simulink model "tpi2series2parallel"  (R2017b)
settings: Solver=ode8  StartTime=0.0  StopTime=0.1  FixedStep=1e-6  MaxStep=1e-4  RelTol=1e-3
values from neighbouring files (symbols this model uses):
  dcin = 547.66    [tpi2parallelrunner.m]    (also in tpi2seriesrunner.m; tpireloadedrunner.m)
  Ef = 154.55/2    (= 77.275)    [tpi2seriesrunner.m]    (also in tpireloadedrunner.m)
  fdclinkcap = 100e-6    (= 0.0001)    [tpi2parallelrunner.m]    (also in tpi2seriesrunner.m; tpireloadedrunner.m = 0.01)
  fdclinkres = 1e-6    (= 1e-06)    [tpi2parallelrunner.m]    (also in tpi2seriesrunner.m; tpireloadedrunner.m)
  FLload = FXload/freffreq    [tpi2parallelrunner.m]    (also in tpi2seriesrunner.m; tpireloadedrunner.m)
  fma = 0.9    [tpi2parallelrunner.m]    (also in tpi2seriesrunner.m; tpireloadedrunner.m)
  freffreq = 2*pi*50    (= 314.159265359)    [tpi2parallelrunner.m]    (also in tpi2seriesrunner.m; tpireloadedrunner.m)
  FRload = FZload*Load_Power_Factor    [tpi2parallelrunner.m]    (also in tpi2seriesrunner.m = n*FZload*Load_Power_Factor; tpireloadedrunner.m = n*FZload*Load_Power_Factor)
  Rin = 1    [tpi2parallelrunner.m]    (also in tpi2seriesrunner.m; tpireloadedrunner.m)
  sdclinkcap = 100e-6    (= 0.0001)    [tpi2seriesrunner.m]    (also in tpireloadedrunner.m = 0.01)
  sdclinkres = 1e-6    (= 1e-06)    [tpi2seriesrunner.m]    (also in tpireloadedrunner.m)
  SLload = SXload/sreffreq    [tpi2parallelrunner.m]    (also in tpi2seriesrunner.m; tpireloadedrunner.m)
  sma = 0.9    [tpi2parallelrunner.m]    (also in tpi2seriesrunner.m; tpireloadedrunner.m)
  sreffreq = 2*pi*50    (= 314.159265359)    [tpi2parallelrunner.m]    (also in tpi2seriesrunner.m; tpireloadedrunner.m)
  SRload = SZload*Load_Power_Factor    [tpi2parallelrunner.m]    (also in tpi2seriesrunner.m = n*SZload*Load_Power_Factor; tpireloadedrunner.m = n*SZload*Load_Power_Factor)
undefined symbols (not defined in the file or in its folder): fdclink1cap
libraries: powerlib x82, simulink x12, powerlib_meascontrol x10, dspstat3 x9
settings Model: Creator=Orhun  LastModifiedBy=Orhun
settings SolverCC: ZeroCrossAlgorithm=Adaptive
settings DebuggingCC: MaxConsecutiveZCsMsg=none

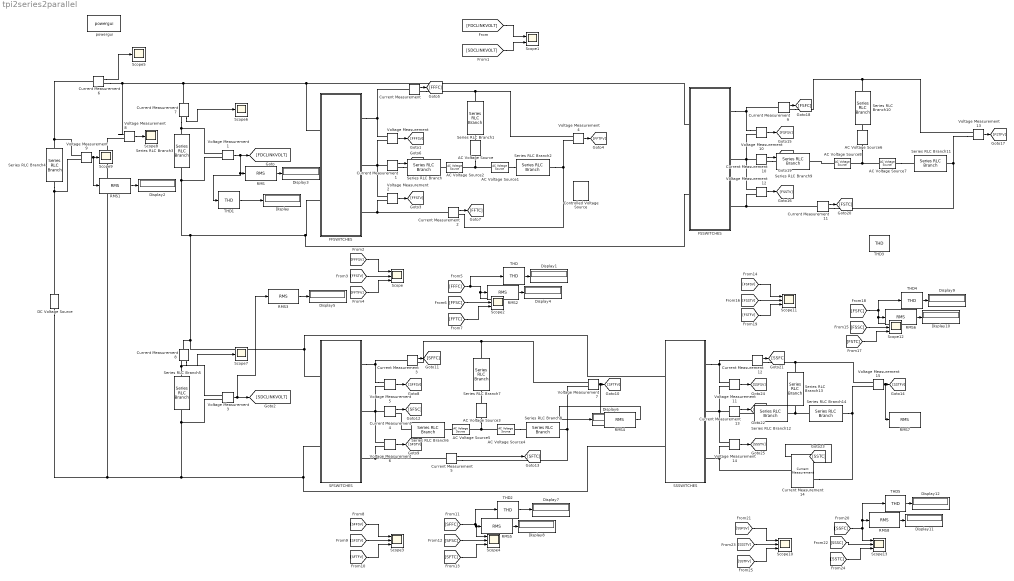
== system tpi2series2parallel ==
  AC Voltage Source : powerlib/Electrical Sources/AC Voltage Source  Amplitude=Ef*sqrt(2)  Phase=0  Frequency=freffreq  SampleTime=0  Measurements=None  BusType=swing  Pref=10e3  Qref=0  Qmin=-inf  Qmax=+inf
  AC Voltage Source1 : powerlib/Electrical Sources/AC Voltage Source  Amplitude=Ef*sqrt(2)  Phase=-2*pi/3  Frequency=freffreq  SampleTime=0  Measurements=None  BusType=swing  Pref=10e3  Qref=0  Qmin=-inf  Qmax=+inf
  AC Voltage Source2 : powerlib/Electrical Sources/AC Voltage Source  Amplitude=Ef*sqrt(2)  Phase=2*pi/3  Frequency=freffreq  SampleTime=0  Measurements=None  BusType=swing  Pref=10e3  Qref=0  Qmin=-inf  Qmax=+inf
  AC Voltage Source3 : powerlib/Electrical Sources/AC Voltage Source  Amplitude=Ef*sqrt(2)  Phase=0  Frequency=sreffreq  SampleTime=0  Measurements=None  BusType=swing  Pref=10e3  Qref=0  Qmin=-inf  Qmax=+inf
  AC Voltage Source4 : powerlib/Electrical Sources/AC Voltage Source  Amplitude=Ef*sqrt(2)  Phase=-2*pi/3  Frequency=sreffreq  SampleTime=0  Measurements=None  BusType=swing  Pref=10e3  Qref=0  Qmin=-inf  Qmax=+inf
  AC Voltage Source5 : powerlib/Electrical Sources/AC Voltage Source  Amplitude=Ef*sqrt(2)  Phase=2*pi/3  Frequency=sreffreq  SampleTime=0  Measurements=None  BusType=swing  Pref=10e3  Qref=0  Qmin=-inf  Qmax=+inf
  AC Voltage Source6 : powerlib/Electrical Sources/AC Voltage Source  Amplitude=Ef*sqrt(2)  Phase=0  Frequency=freffreq  SampleTime=0  Measurements=None  BusType=swing  Pref=10e3  Qref=0  Qmin=-inf  Qmax=+inf
  AC Voltage Source7 : powerlib/Electrical Sources/AC Voltage Source  Amplitude=Ef*sqrt(2)  Phase=-2*pi/3  Frequency=freffreq  SampleTime=0  Measurements=None  BusType=swing  Pref=10e3  Qref=0  Qmin=-inf  Qmax=+inf
  AC Voltage Source8 : powerlib/Electrical Sources/AC Voltage Source  Amplitude=Ef*sqrt(2)  Phase=2*pi/3  Frequency=freffreq  SampleTime=0  Measurements=None  BusType=swing  Pref=10e3  Qref=0  Qmin=-inf  Qmax=+inf
  Controlled Voltage Source : powerlib/Electrical Sources/Controlled Voltage Source  Initialize=on  Source_Type=AC  Amplitude=0  Phase=0  Frequency=0  Measurements=None
  Current Measurement{,1..14} (15 alike) : powerlib/Measurements/Current Measurement  PhasorSimulation=off  OutputType=Complex  PSBequivalent=0
  DC Voltage Source : powerlib/Electrical Sources/DC Voltage Source  Amplitude=dcin  Measurements=None
  Display{,1..12} (13 alike) : Display
  FFSWITCHES : Subsystem
  FSSWITCHES : Subsystem
  RMS : dspstat3/RMS  run=on  directionMode=Each column  dimension=1  InputProcessing=Columns as channels (frame based)  reset_popup=None
  RMS1 : dspstat3/RMS  run=off  directionMode=Each column  dimension=1  InputProcessing=Columns as channels (frame based)  reset_popup=None
  RMS{2,4..8} (6 alike) : dspstat3/RMS  run=on  directionMode=Entire input  dimension=1  InputProcessing=Columns as channels (frame based)  reset_popup=None
  RMS3 : dspstat3/RMS  run=off  directionMode=Each column  dimension=1  InputProcessing=Columns as channels (frame based)  reset_popup=None
  SFSWITCHES : Subsystem
  SSSWITCHES : Subsystem
  Scope{,2..4,10..13} (8 alike) : Scope  NumInputPorts=3
  Scope1 : Scope  NumInputPorts=2
  Scope{5..9} (5 alike) : Scope
  Series RLC Branch{,1..2,9..11} (6 alike) : powerlib/Elements/Series RLC Branch  LConnTagsString=__new0  RConnTagsString=__new0  BranchType=RL  Resistance=FRload  Inductance=FLload  SetiL0=off  InitialCurrent=0  Capacitance=0  Setx0=off  InitialVoltage=0  Measurements=None
  Series RLC Branch{6..8,12..14} (6 alike) : powerlib/Elements/Series RLC Branch  LConnTagsString=__new0  RConnTagsString=__new0  BranchType=RL  Resistance=SRload  Inductance=SLload  SetiL0=off  InitialCurrent=0  Capacitance=0  Setx0=off  InitialVoltage=0  Measurements=None
  Series RLC Branch3 : powerlib/Elements/Series RLC Branch  LConnTagsString=__new0  RConnTagsString=__new0  BranchType=C  Resistance=fdclinkres  Inductance=0  SetiL0=off  InitialCurrent=0  Capacitance=fdclinkcap  Setx0=off  InitialVoltage=dcin/2  Measurements=None
  Series RLC Branch4 : powerlib/Elements/Series RLC Branch  LConnTagsString=__new0  RConnTagsString=__new0  BranchType=R  Resistance=Rin  Inductance=0  SetiL0=off  InitialCurrent=0  Capacitance=fdclink1cap  Setx0=off  InitialVoltage=0  Measurements=None
  Series RLC Branch5 : powerlib/Elements/Series RLC Branch  LConnTagsString=__new0  RConnTagsString=__new0  BranchType=C  Resistance=sdclinkres  Inductance=0  SetiL0=off  InitialCurrent=0  Capacitance=sdclinkcap  Setx0=off  InitialVoltage=dcin/2  Measurements=None
  THD{,1..5} (6 alike) : powerlib_meascontrol/Measurements/THD  Freq=50  Ts=0
  Voltage Measurement{,1..15} (16 alike) : powerlib/Measurements/Voltage Measurement  PhasorSimulation=off  OutputType=Complex  PSBequivalent=0
  powergui : powerlib/powergui  Priority=1  SimulationMode=Discrete  SampleTime=1e-6  frequency=60  Iterations=50  frequencyindice=0  Pbase=100e6  ErrMax=1e-4  UnitsV=kV  UnitsW=MW  buscounter=0  FunctionMessages=on  echomessages=off  EnableUseOfTLC=off  CurrentSourceSwitches=off  DisableSnubberDevices=off  DisableRonSwitches=off  DisableVfSwitches=off  DisplayEquations=off  SolverType=Tustin/Backward Euler (TBE)  Interpol=off  ExternalGateDelay=off  methode=off  Ts=100  x0status=blocks  SPID=off  SwTol=0  HookPort=off  RestoreLinks=warning  ResistiveCurrentMeasurement=off  Frange=[0:2:500]  Ylog=off  Xlog=on  ShowGrid=off  save=off  variable=ZData  structure=0  ZoomFFT=off  StartTime=0.0  cycles=1  DisplayStyle=1  fundamental=60  FreqAxis=off  MaxFrequency=1000  frequencyindicesteady=1  RmsSteady=1  display=off
  wires:
  Voltage Measurement1/1 -> RMS/1, THD1/1, [FDCLINKVOLT]
  Voltage Measurement3/1 -> RMS3/1, [SDCLINKVOLT]
  [FDCLINKVOLT] -> Scope1/1
  [SDCLINKVOLT] -> Scope1/2
  Voltage Measurement/1 -> [FFFSV]
  Voltage Measurement2/1 -> [FFSTV]
  Voltage Measurement4/1 -> [FFTFV]
  Current Measurement/1 -> [FFFC]
  Current Measurement1/1 -> [FFSC]
  Current Measurement2/1 -> [FFTC]
  [FFFSV] -> Scope/1
  [FFSTV] -> Scope/2
  [FFTFV] -> Scope/3
  [FFFC] -> THD/1, RMS2/1, Scope2/1
  [SFSTV] -> Scope3/2
  [SFTC] -> Scope4/3
  [SFTFV] -> Scope3/3
  [SFSC] -> Scope4/2
  [SFFSV] -> Scope3/1
  [SFFC] -> THD2/1, RMS5/1, Scope4/1
  Current Measurement3/1 -> [SFFC]
  Current Measurement4/1 -> [SFSC]
  Voltage Measurement5/1 -> [SFFSV]
  Voltage Measurement6/1 -> [SFSTV]
  Current Measurement5/1 -> [SFTC]
  Voltage Measurement7/1 -> RMS4/1, [SFTFV]
  Current Measurement6/1 -> Scope5/1
  THD1/1 -> Display/1
  Current Measurement7/1 -> Scope6/1
  Current Measurement8/1 -> Scope7/1
  THD/1 -> Display1/1
  Voltage Measurement8/1 -> Scope8/1
  Voltage Measurement9/1 -> RMS1/1, Scope9/1
  RMS1/1 -> Display2/1
  RMS/1 -> Display3/1
  RMS2/1 -> Display4/1
  RMS3/1 -> Display5/1
  RMS4/1 -> Display6/1
  [FFSC] -> Scope2/2
  [FFTC] -> Scope2/3
  THD2/1 -> Display7/1
  Current Measurement9/1 -> [FSFC]
  Current Measurement11/1 -> [FSTC]
  Voltage Measurement10/1 -> [FSFSV]
  Current Measurement10/1 -> [FSSC]
  Voltage Measurement13/1 -> [FSTFV]
  Voltage Measurement12/1 -> [FSSTV]
  [FSFSV] -> Scope11/1
  RMS6/1 -> Display10/1
  THD4/1 -> Display9/1
  [FSTC] -> Scope12/3
  [FSFC] -> THD4/1, RMS6/1, Scope12/1
  Voltage Measurement15/1 -> RMS7/1, [SSTFV]
  Voltage Measurement11/1 -> [SSFSV]
  Current Measurement14/1 -> [SSTC]
  Voltage Measurement14/1 -> [SSSTV]
  Current Measurement12/1 -> [SSFC]
  Current Measurement13/1 -> [SSSC]
  [SSFSV] -> Scope10/1
  [SSSTV] -> Scope10/2
  [SSTFV] -> Scope10/3
  [SSSC] -> Scope13/2
  [SSFC] -> RMS8/1, THD5/1, Scope13/1
  RMS8/1 -> Display11/1
  [SSTC] -> Scope13/3
  THD5/1 -> Display12/1
  [FSSC] -> Scope12/2
  [FSTFV] -> Scope11/3
  [FSSTV] -> Scope11/2
  RMS5/1 -> Display8/1
  connections:
  Current Measurement6/RConn1 -- Voltage Measurement8/LConn1 -- Current Measurement7/LConn1 -- FSSWITCHES/LConn1 -- FFSWITCHES/LConn1
  Voltage Measurement1/LConn2 -- FSSWITCHES/LConn2 -- FFSWITCHES/LConn2 -- SSSWITCHES/LConn1 -- SFSWITCHES/LConn1 -- Current Measurement8/LConn1 -- Series RLC Branch3/RConn1
  Series RLC Branch4/RConn1 -- Voltage Measurement9/LConn2 -- DC Voltage Source/RConn1
  Voltage Measurement3/LConn2 -- Voltage Measurement8/LConn2 -- DC Voltage Source/LConn1 -- SSSWITCHES/LConn2 -- SFSWITCHES/LConn2 -- Series RLC Branch5/RConn1
  FFSWITCHES/RConn1 -- Current Measurement/LConn1 -- Voltage Measurement/LConn1
  FFSWITCHES/RConn2 -- Current Measurement1/LConn1 -- Voltage Measurement2/LConn1 -- Voltage Measurement/LConn2
  Series RLC Branch2/LConn1 -- Current Measurement2/RConn1 -- Voltage Measurement4/LConn1
  Current Measurement/RConn1 -- Series RLC Branch1/RConn1 -- Voltage Measurement4/LConn2
  Current Measurement1/RConn1 -- Series RLC Branch/RConn1
  Voltage Measurement2/LConn2 -- Current Measurement2/LConn1 -- FFSWITCHES/RConn3
  Current Measurement3/RConn1 -- Series RLC Branch7/RConn1 -- Voltage Measurement7/LConn2
  Voltage Measurement5/LConn1 -- SFSWITCHES/RConn1 -- Current Measurement3/LConn1
  Voltage Measurement5/LConn2 -- SFSWITCHES/RConn2 -- Current Measurement4/LConn1 -- Voltage Measurement6/LConn1
  Series RLC Branch8/LConn1 -- Voltage Measurement7/LConn1 -- Current Measurement5/RConn1
  Voltage Measurement6/LConn2 -- Current Measurement5/LConn1 -- SFSWITCHES/RConn3
  Series RLC Branch6/RConn1 -- Current Measurement4/RConn1
  Current Measurement6/LConn1 -- Voltage Measurement9/LConn1 -- Series RLC Branch4/LConn1
  Voltage Measurement1/LConn1 -- Current Measurement7/RConn1 -- Series RLC Branch3/LConn1
  Series RLC Branch5/LConn1 -- Voltage Measurement3/LConn1 -- Current Measurement8/RConn1
  FSSWITCHES/RConn3 -- Voltage Measurement12/LConn2 -- Current Measurement11/LConn1
  Voltage Measurement10/LConn1 -- FSSWITCHES/RConn1 -- Current Measurement9/LConn1
  Voltage Measurement13/LConn1 -- Series RLC Branch11/LConn1 -- Current Measurement11/RConn1
  Current Measurement9/RConn1 -- Voltage Measurement13/LConn2 -- Series RLC Branch10/RConn1
  Voltage Measurement10/LConn2 -- FSSWITCHES/RConn2 -- Current Measurement10/LConn1 -- Voltage Measurement12/LConn1
  Current Measurement10/RConn1 -- Series RLC Branch9/RConn1
  Current Measurement12/LConn1 -- Voltage Measurement11/LConn1 -- SSSWITCHES/RConn1
  Current Measurement14/RConn1 -- Voltage Measurement15/LConn1 -- Series RLC Branch14/LConn1
  SSSWITCHES/RConn3 -- Voltage Measurement14/LConn2 -- Current Measurement14/LConn1
  Series RLC Branch12/LConn1 -- Series RLC Branch14/RConn1 -- Series RLC Branch13/LConn1
  Voltage Measurement14/LConn1 -- Voltage Measurement11/LConn2 -- SSSWITCHES/RConn2 -- Current Measurement13/LConn1
  Voltage Measurement15/LConn2 -- Current Measurement12/RConn1 -- Series RLC Branch13/RConn1
  Series RLC Branch12/RConn1 -- Current Measurement13/RConn1
  AC Voltage Source/RConn1 -- Series RLC Branch1/LConn1
  AC Voltage Source1/RConn1 -- Series RLC Branch2/RConn1
  AC Voltage Source2/RConn1 -- Series RLC Branch/LConn1
  AC Voltage Source1/LConn1 -- AC Voltage Source/LConn1 -- AC Voltage Source2/LConn1
  AC Voltage Source4/LConn1 -- AC Voltage Source3/LConn1 -- AC Voltage Source5/LConn1
  AC Voltage Source3/RConn1 -- Series RLC Branch7/LConn1
  Series RLC Branch6/LConn1 -- AC Voltage Source5/RConn1
  AC Voltage Source4/RConn1 -- Series RLC Branch8/RConn1
  AC Voltage Source7/LConn1 -- AC Voltage Source6/LConn1 -- AC Voltage Source8/LConn1
  AC Voltage Source6/RConn1 -- Series RLC Branch10/LConn1
  AC Voltage Source8/RConn1 -- Series RLC Branch9/LConn1
  AC Voltage Source7/RConn1 -- Series RLC Branch11/RConn1

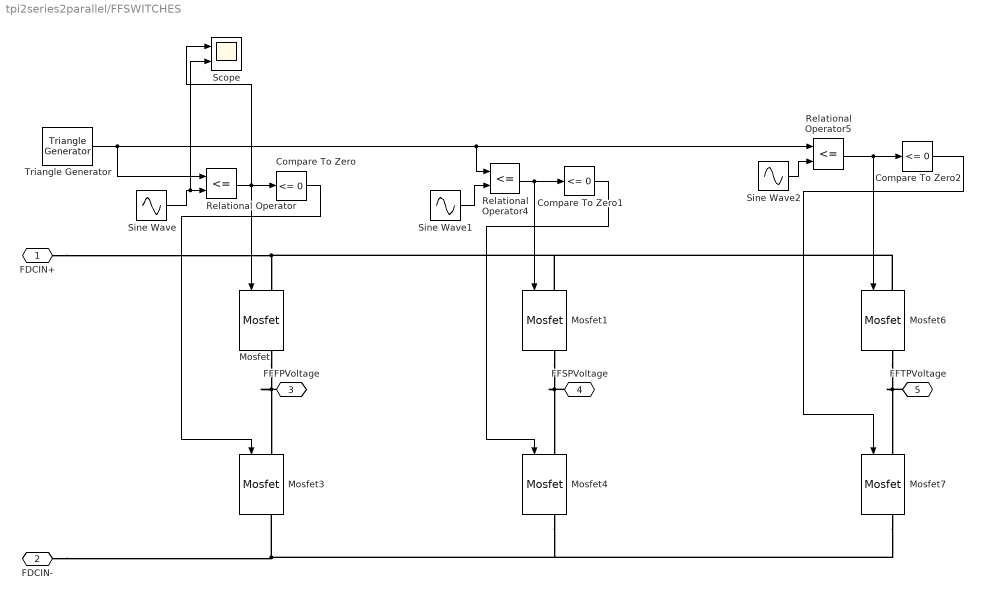
== system tpi2series2parallel/FFSWITCHES ==
  Compare To Zero : simulink/Logic and Bit Operations/Compare To Zero  relop=<=  OutDataTypeStr=boolean
  Compare To Zero1 : simulink/Logic and Bit Operations/Compare To Zero  relop=<=  OutDataTypeStr=boolean
  Compare To Zero2 : simulink/Logic and Bit Operations/Compare To Zero  relop=<=  OutDataTypeStr=boolean
  Mosfet{,1,3..4,6..7} (6 alike) : powerlib/Power Electronics/Mosfet  Ron=2e-3  Lon=0  Rd=0.01  Vfd=0  IC=0  Rs=1e5  Cs=inf  Measurements=on
  Relational Operator : RelationalOperator  Operator=<=  OutDataTypeStr=boolean  RndMeth=Simplest
  Relational Operator4 : RelationalOperator  Operator=<=  OutDataTypeStr=boolean  RndMeth=Simplest
  Relational Operator5 : RelationalOperator  Operator=<=  OutDataTypeStr=boolean  RndMeth=Simplest
  Scope : Scope  NumInputPorts=2
  Sine Wave : Sin  Amplitude=fma  Frequency=freffreq  SampleTime=0
  Sine Wave1 : Sin  Amplitude=fma  Frequency=freffreq  Phase=2*pi/3  SampleTime=0
  Sine Wave2 : Sin  Amplitude=fma  Frequency=freffreq  Phase=4*pi/3  SampleTime=0
  Triangle Generator : powerlib_meascontrol/Pulse & Signal Generators/Triangle Generator  Freq=fswfreq  Phase=90  Ts=1e-6
  FDCIN+ : PMIOPort  Port=1  Side=Left
  FDCIN- : PMIOPort  Port=2  Side=Left
  FFFPVoltage : PMIOPort  Port=3  Side=Right
  FFSPVoltage : PMIOPort  Port=4  Side=Right
  FFTPVoltage : PMIOPort  Port=5  Side=Right
  wires:
  Sine Wave/1 -> Scope/2, Relational Operator/2
  Triangle Generator/1 -> Relational Operator5/1, Relational Operator4/1, Relational Operator/1
  Relational Operator4/1 -> Mosfet1/1, Compare To Zero1/1
  Sine Wave2/1 -> Relational Operator5/2
  Sine Wave1/1 -> Relational Operator4/2
  Relational Operator/1 -> Mosfet/1, Scope/1, Compare To Zero/1
  Compare To Zero/1 -> Mosfet3/1
  Compare To Zero1/1 -> Mosfet4/1
  Compare To Zero2/1 -> Mosfet7/1
  Relational Operator5/1 -> Mosfet6/1, Compare To Zero2/1
  connections:
  Mosfet6/RConn1 -- FFTPVoltage/RConn1 -- Mosfet7/LConn1
  Mosfet/RConn1 -- FFFPVoltage/RConn1 -- Mosfet3/LConn1
  Mosfet1/RConn1 -- FFSPVoltage/RConn1 -- Mosfet4/LConn1
  FDCIN+/RConn1 -- Mosfet6/LConn1 -- Mosfet1/LConn1 -- Mosfet/LConn1
  FDCIN-/RConn1 -- Mosfet4/RConn1 -- Mosfet7/RConn1 -- Mosfet3/RConn1

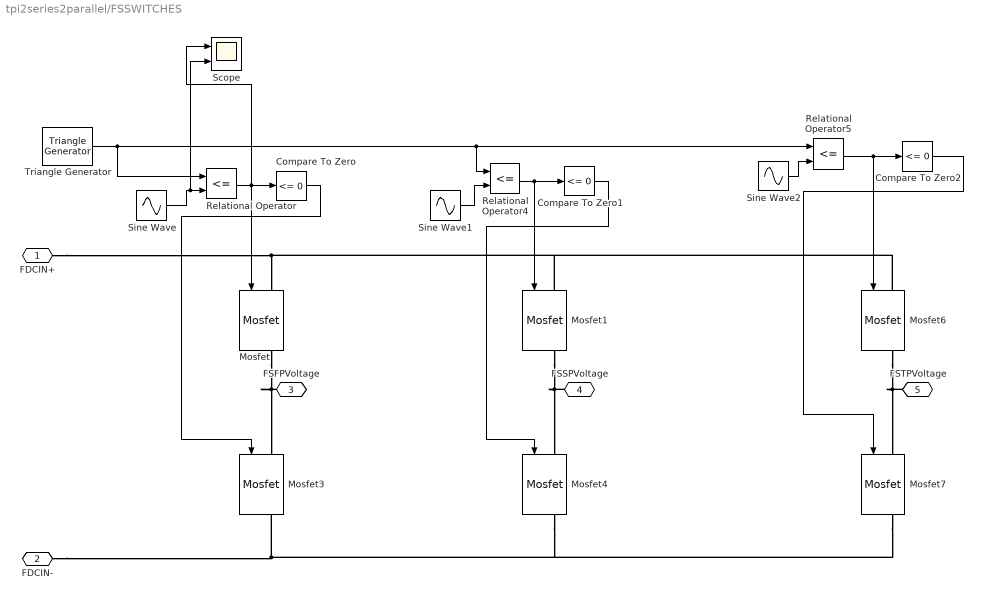
== system tpi2series2parallel/FSSWITCHES ==
  Compare To Zero : simulink/Logic and Bit Operations/Compare To Zero  relop=<=  OutDataTypeStr=boolean
  Compare To Zero1 : simulink/Logic and Bit Operations/Compare To Zero  relop=<=  OutDataTypeStr=boolean
  Compare To Zero2 : simulink/Logic and Bit Operations/Compare To Zero  relop=<=  OutDataTypeStr=boolean
  Mosfet{,1,3..4,6..7} (6 alike) : powerlib/Power Electronics/Mosfet  Ron=2e-3  Lon=0  Rd=0.01  Vfd=0  IC=0  Rs=1e5  Cs=inf  Measurements=on
  Relational Operator : RelationalOperator  Operator=<=  OutDataTypeStr=boolean  RndMeth=Simplest
  Relational Operator4 : RelationalOperator  Operator=<=  OutDataTypeStr=boolean  RndMeth=Simplest
  Relational Operator5 : RelationalOperator  Operator=<=  OutDataTypeStr=boolean  RndMeth=Simplest
  Scope : Scope  NumInputPorts=2
  Sine Wave : Sin  Amplitude=fma  Frequency=freffreq  SampleTime=0
  Sine Wave1 : Sin  Amplitude=fma  Frequency=freffreq  Phase=2*pi/3  SampleTime=0
  Sine Wave2 : Sin  Amplitude=fma  Frequency=freffreq  Phase=4*pi/3  SampleTime=0
  Triangle Generator : powerlib_meascontrol/Pulse & Signal Generators/Triangle Generator  Freq=fswfreq  Phase=90  Ts=1e-6
  FDCIN+ : PMIOPort  Port=1  Side=Left
  FDCIN- : PMIOPort  Port=2  Side=Left
  FSFPVoltage : PMIOPort  Port=3  Side=Right
  FSSPVoltage : PMIOPort  Port=4  Side=Right
  FSTPVoltage : PMIOPort  Port=5  Side=Right
  wires:
  Sine Wave/1 -> Scope/2, Relational Operator/2
  Triangle Generator/1 -> Relational Operator5/1, Relational Operator4/1, Relational Operator/1
  Relational Operator4/1 -> Mosfet1/1, Compare To Zero1/1
  Sine Wave2/1 -> Relational Operator5/2
  Sine Wave1/1 -> Relational Operator4/2
  Relational Operator/1 -> Mosfet/1, Scope/1, Compare To Zero/1
  Compare To Zero/1 -> Mosfet3/1
  Compare To Zero1/1 -> Mosfet4/1
  Compare To Zero2/1 -> Mosfet7/1
  Relational Operator5/1 -> Mosfet6/1, Compare To Zero2/1
  connections:
  Mosfet6/RConn1 -- FSTPVoltage/RConn1 -- Mosfet7/LConn1
  Mosfet/RConn1 -- FSFPVoltage/RConn1 -- Mosfet3/LConn1
  Mosfet1/RConn1 -- FSSPVoltage/RConn1 -- Mosfet4/LConn1
  FDCIN+/RConn1 -- Mosfet6/LConn1 -- Mosfet1/LConn1 -- Mosfet/LConn1
  FDCIN-/RConn1 -- Mosfet4/RConn1 -- Mosfet7/RConn1 -- Mosfet3/RConn1

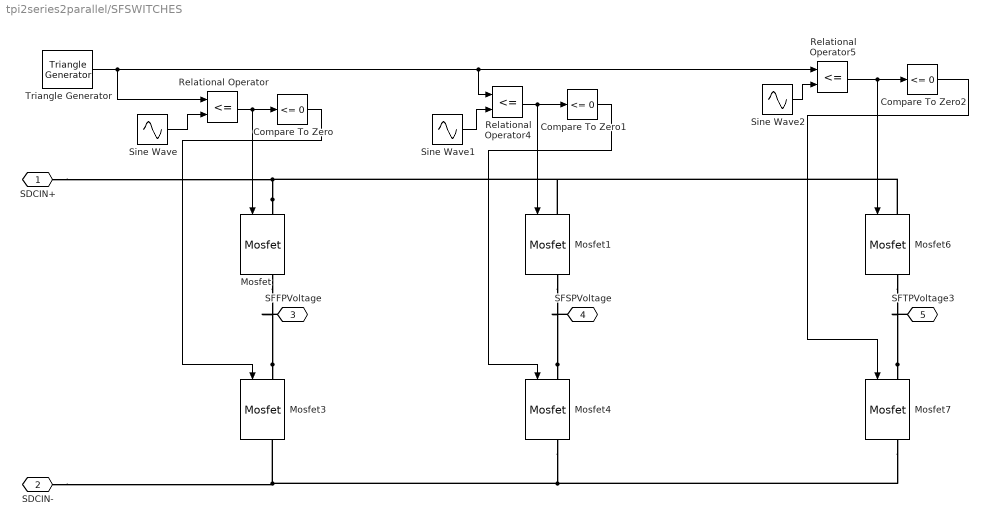
== system tpi2series2parallel/SFSWITCHES ==
  Compare To Zero : simulink/Logic and Bit Operations/Compare To Zero  relop=<=  OutDataTypeStr=boolean
  Compare To Zero1 : simulink/Logic and Bit Operations/Compare To Zero  relop=<=  OutDataTypeStr=boolean
  Compare To Zero2 : simulink/Logic and Bit Operations/Compare To Zero  relop=<=  OutDataTypeStr=boolean
  Mosfet{,1,3..4,6..7} (6 alike) : powerlib/Power Electronics/Mosfet  Ron=2e-3  Lon=0  Rd=0.01  Vfd=0  IC=0  Rs=1e5  Cs=inf  Measurements=on
  Relational Operator : RelationalOperator  Operator=<=  OutDataTypeStr=boolean  RndMeth=Simplest
  Relational Operator4 : RelationalOperator  Operator=<=  OutDataTypeStr=boolean  RndMeth=Simplest
  Relational Operator5 : RelationalOperator  Operator=<=  OutDataTypeStr=boolean  RndMeth=Simplest
  Sine Wave : Sin  Amplitude=sma  Frequency=sreffreq  SampleTime=0
  Sine Wave1 : Sin  Amplitude=sma  Frequency=sreffreq  Phase=2*pi/3  SampleTime=0
  Sine Wave2 : Sin  Amplitude=fma  Frequency=sreffreq  Phase=4*pi/3  SampleTime=0
  Triangle Generator : powerlib_meascontrol/Pulse & Signal Generators/Triangle Generator  Freq=sswfreq  Phase=270  Ts=1e-6
  SDCIN+ : PMIOPort  Port=1  Side=Left
  SDCIN- : PMIOPort  Port=2  Side=Left
  SFFPVoltage : PMIOPort  Port=3  Side=Right
  SFSPVoltage : PMIOPort  Port=4  Side=Right
  SFTPVoltage3 : PMIOPort  Port=5  Side=Right
  wires:
  Sine Wave/1 -> Relational Operator/2
  Triangle Generator/1 -> Relational Operator5/1, Relational Operator4/1, Relational Operator/1
  Relational Operator4/1 -> Mosfet1/1, Compare To Zero1/1
  Sine Wave2/1 -> Relational Operator5/2
  Sine Wave1/1 -> Relational Operator4/2
  Relational Operator/1 -> Compare To Zero/1, Mosfet/1
  Compare To Zero/1 -> Mosfet3/1
  Compare To Zero1/1 -> Mosfet4/1
  Compare To Zero2/1 -> Mosfet7/1
  Relational Operator5/1 -> Mosfet6/1, Compare To Zero2/1
  connections:
  Mosfet7/LConn1 -- Mosfet6/RConn1 -- SFTPVoltage3/RConn1
  Mosfet3/LConn1 -- Mosfet/RConn1 -- SFFPVoltage/RConn1
  Mosfet4/LConn1 -- Mosfet1/RConn1 -- SFSPVoltage/RConn1
  Mosfet/LConn1 -- SDCIN+/RConn1 -- Mosfet6/LConn1 -- Mosfet1/LConn1
  Mosfet4/RConn1 -- Mosfet3/RConn1 -- SDCIN-/RConn1 -- Mosfet7/RConn1

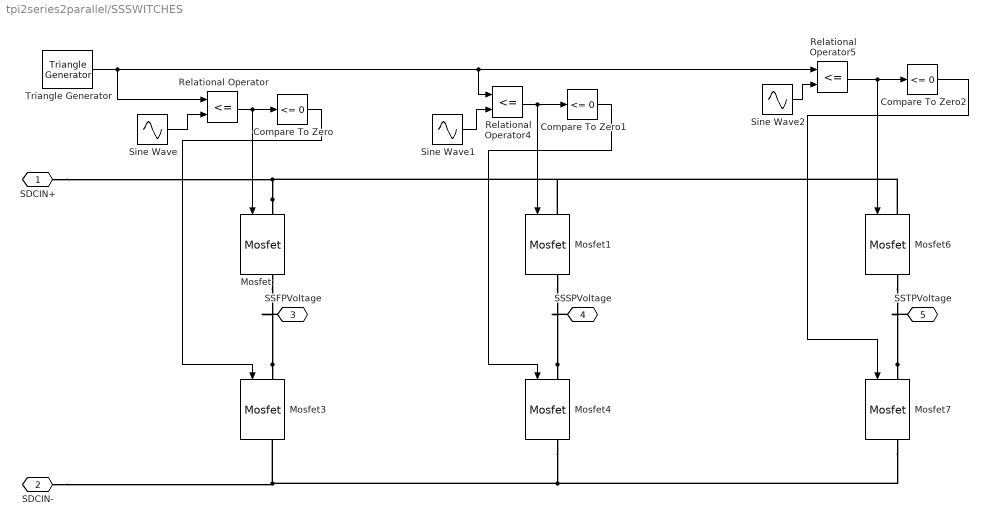
== system tpi2series2parallel/SSSWITCHES ==
  Compare To Zero : simulink/Logic and Bit Operations/Compare To Zero  relop=<=  OutDataTypeStr=boolean
  Compare To Zero1 : simulink/Logic and Bit Operations/Compare To Zero  relop=<=  OutDataTypeStr=boolean
  Compare To Zero2 : simulink/Logic and Bit Operations/Compare To Zero  relop=<=  OutDataTypeStr=boolean
  Mosfet{,1,3..4,6..7} (6 alike) : powerlib/Power Electronics/Mosfet  Ron=2e-3  Lon=0  Rd=0.01  Vfd=0  IC=0  Rs=1e5  Cs=inf  Measurements=on
  Relational Operator : RelationalOperator  Operator=<=  OutDataTypeStr=boolean  RndMeth=Simplest
  Relational Operator4 : RelationalOperator  Operator=<=  OutDataTypeStr=boolean  RndMeth=Simplest
  Relational Operator5 : RelationalOperator  Operator=<=  OutDataTypeStr=boolean  RndMeth=Simplest
  Sine Wave : Sin  Amplitude=sma  Frequency=sreffreq  SampleTime=0
  Sine Wave1 : Sin  Amplitude=sma  Frequency=sreffreq  Phase=2*pi/3  SampleTime=0
  Sine Wave2 : Sin  Amplitude=fma  Frequency=sreffreq  Phase=4*pi/3  SampleTime=0
  Triangle Generator : powerlib_meascontrol/Pulse & Signal Generators/Triangle Generator  Freq=sswfreq  Phase=270  Ts=1e-6
  SDCIN+ : PMIOPort  Port=1  Side=Left
  SDCIN- : PMIOPort  Port=2  Side=Left
  SSFPVoltage : PMIOPort  Port=3  Side=Right
  SSSPVoltage : PMIOPort  Port=4  Side=Right
  SSTPVoltage : PMIOPort  Port=5  Side=Right
  wires:
  Sine Wave/1 -> Relational Operator/2
  Triangle Generator/1 -> Relational Operator5/1, Relational Operator4/1, Relational Operator/1
  Relational Operator4/1 -> Mosfet1/1, Compare To Zero1/1
  Sine Wave2/1 -> Relational Operator5/2
  Sine Wave1/1 -> Relational Operator4/2
  Relational Operator/1 -> Compare To Zero/1, Mosfet/1
  Compare To Zero/1 -> Mosfet3/1
  Compare To Zero1/1 -> Mosfet4/1
  Compare To Zero2/1 -> Mosfet7/1
  Relational Operator5/1 -> Mosfet6/1, Compare To Zero2/1
  connections:
  Mosfet7/LConn1 -- Mosfet6/RConn1 -- SSTPVoltage/RConn1
  Mosfet3/LConn1 -- Mosfet/RConn1 -- SSFPVoltage/RConn1
  Mosfet4/LConn1 -- Mosfet1/RConn1 -- SSSPVoltage/RConn1
  Mosfet/LConn1 -- SDCIN+/RConn1 -- Mosfet6/LConn1 -- Mosfet1/LConn1
  Mosfet4/RConn1 -- Mosfet3/RConn1 -- SDCIN-/RConn1 -- Mosfet7/RConn1
